simulink model "hw1_simulink"  (R2021b)
settings: Solver=VariableStepAuto  StartTime=0.0  StopTime=10.0  RelTol=1e-3
settings Model: Creator=A  LastModifiedBy=A

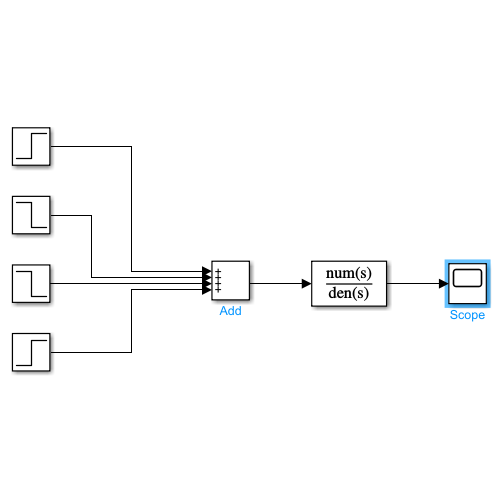
[thumbnail: Simulink's stored preview of the top-level diagram]
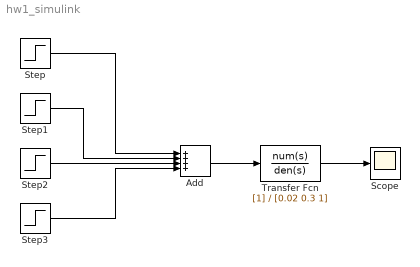
== system hw1_simulink ==
  Add : Sum  Inputs=++++
  Scope : Scope
  Step : Step  Time=2  SampleTime=0
  Step1 : Step  Time=4  Before=1  After=0  SampleTime=0
  Step2 : Step  Time=6  After=-1  SampleTime=0
  Step3 : Step  Time=8  Before=-1  After=0  SampleTime=0
  Transfer Fcn : TransferFcn  Denominator=[0.02 0.3 1]
  wires:
  Step1/1 -> Add/2
  Step/1 -> Add/1
  Step2/1 -> Add/3
  Step3/1 -> Add/4
  Add/1 -> Transfer Fcn/1
  Transfer Fcn/1 -> Scope/1
